simulink model "ecuaciontermodinamica"  (R2022b)
settings: Solver=VariableStepAuto  StartTime=0.0  StopTime=10.0  RelTol=1e-3
settings Model: Creator=gonza  LastModifiedBy=gonza

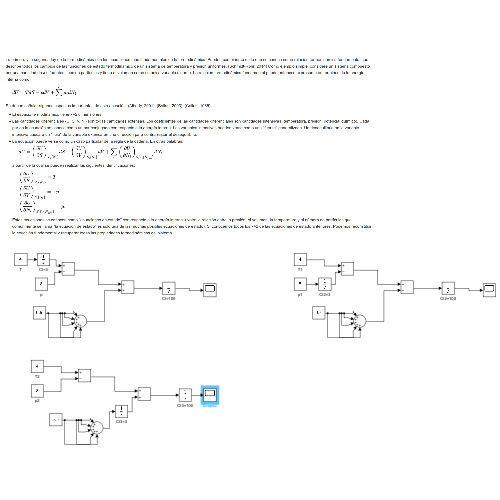
[thumbnail: Simulink's stored preview of the top-level diagram]
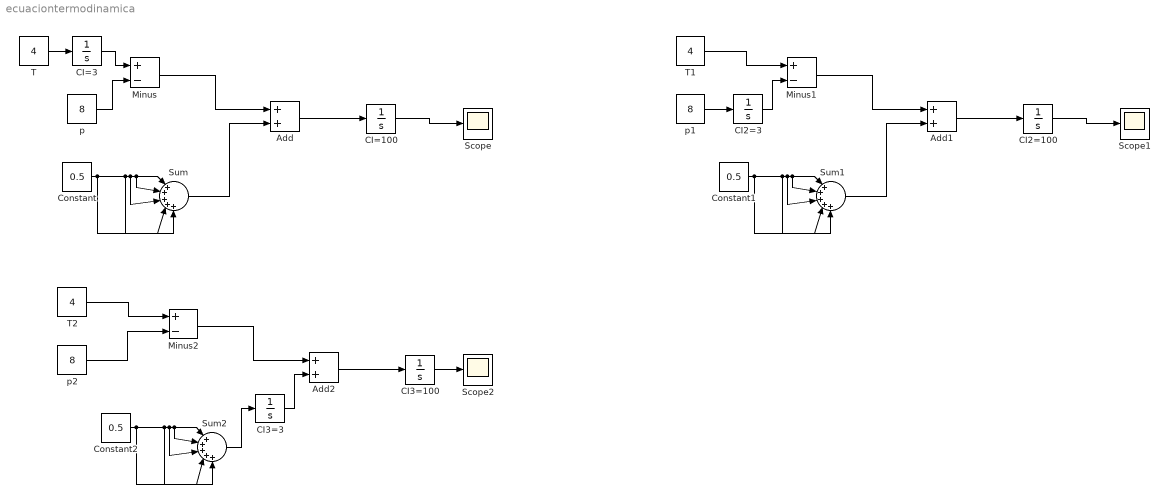
== system ecuaciontermodinamica ==
  Add : Sum
  Add1 : Sum
  Add2 : Sum
  CI2=100 : Integrator  InitialCondition=100
  CI2=3 : Integrator
  CI3=100 : Integrator  InitialCondition=100
  CI3=3 : Integrator
  CI=100 : Integrator  InitialCondition=100
  CI=3 : Integrator  InitialCondition=3
  Constant : Constant  Value=0.5
  Constant1 : Constant  Value=0.5
  Constant2 : Constant  Value=0.5
  Minus : Sum  Inputs=+-
  Minus1 : Sum  Inputs=+-
  Minus2 : Sum  Inputs=+-
  Scope : Scope
  Scope1 : Scope
  Scope2 : Scope
  Sum : Sum  Inputs=|+++++
  Sum1 : Sum  Inputs=|+++++
  Sum2 : Sum  Inputs=|+++++
  T : Constant  Value=4
  T1 : Constant  Value=4
  T2 : Constant  Value=4
  p : Constant  Value=8
  p1 : Constant  Value=8
  p2 : Constant  Value=8
  wires:
  p/1 -> Minus/2
  T/1 -> CI=3/1
  CI=3/1 -> Minus/1
  Constant/1 -> Sum/5, Sum/4, Sum/3, Sum/2, Sum/1
  Minus/1 -> Add/1
  Sum/1 -> Add/2
  Add/1 -> CI=100/1
  CI=100/1 -> Scope/1
  Minus1/1 -> Add1/1
  Sum1/1 -> Add1/2
  Add1/1 -> CI2=100/1
  T1/1 -> Minus1/1
  Constant1/1 -> Sum1/5, Sum1/4, Sum1/3, Sum1/2, Sum1/1
  CI2=100/1 -> Scope1/1
  CI2=3/1 -> Minus1/2
  p1/1 -> CI2=3/1
  Constant2/1 -> Sum2/5, Sum2/4, Sum2/3, Sum2/2, Sum2/1
  Add2/1 -> CI3=100/1
  Minus2/1 -> Add2/1
  T2/1 -> Minus2/1
  p2/1 -> Minus2/2
  CI3=3/1 -> Add2/2
  Sum2/1 -> CI3=3/1
  CI3=100/1 -> Scope2/1
